simulink model "Simulation_invdyn"  (R2022b)
settings: Solver=ode1  StartTime=0.0  StopTime=Tf  FixedStep=t_step  RelTol=1e-3
undefined symbols (not defined in the file or in its folder): F, Im, Kd, Kp, kr, lx, ly, lz, mm, qt, rho, t_step
settings Model: Creator=vincenzo  LastModifiedBy=vincenzo

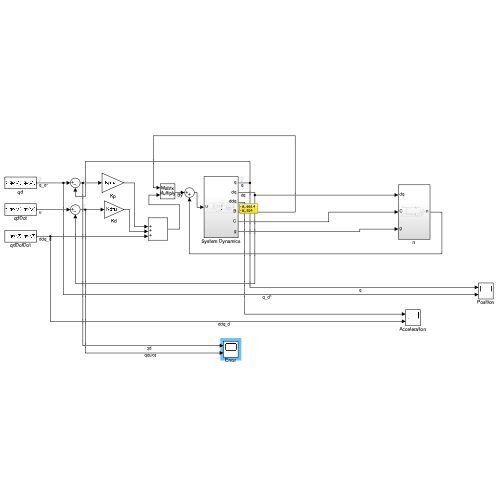
[thumbnail: Simulink's stored preview of the top-level diagram]
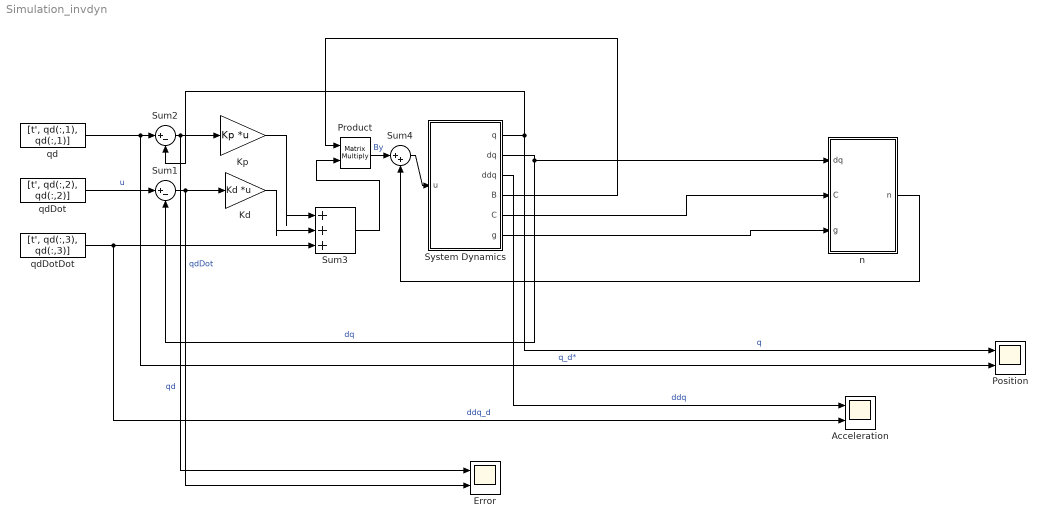
== system Simulation_invdyn ==
  Acceleration : Scope  NumInputPorts=2
  Error : Scope  NumInputPorts=2
  Kd : Gain  Gain=Kd  Multiplication=Matrix(K*u)
  Kp : Gain  Gain=Kp  Multiplication=Matrix(K*u)
  Position : Scope  NumInputPorts=2
  Product : Product  Multiplication=Matrix(*)
  Sum1 : Sum  Inputs=|+-
  Sum2 : Sum  Inputs=|+-
  Sum3 : Sum  Inputs=|+++
  Sum4 : Sum  Inputs=|++
  System Dynamics : Subsystem
  n : Subsystem
  qd : FromWorkspace  VariableName=[t', qd(:,1), qd(:,1)]  OutDataTypeStr=double  SampleTime=t_step
  qdDot : FromWorkspace  VariableName=[t', qd(:,2), qd(:,2)]  OutDataTypeStr=double  SampleTime=t_step
  qdDotDot : FromWorkspace  VariableName=[t', qd(:,3), qd(:,3)]  OutDataTypeStr=double  SampleTime=t_step
  wires:
  System Dynamics/2(dq) -> Sum1/2, n/1(dq)  "dq"
  System Dynamics/4(B) -> Product/1
  System Dynamics/5(C) -> n/2(C)
  System Dynamics/6(g) -> n/3(g)
  qd/1 -> Position/2, Sum2/1  "q_d*"
  Sum2/1 -> Error/1, Kp/1  "qd"
  qdDot/1 -> Sum1/1  "u"
  Sum1/1 -> Error/2, Kd/1  "qdDot"
  System Dynamics/1(q) -> Position/1, Sum2/2  "q"
  Kp/1 -> Sum3/1
  Kd/1 -> Sum3/2
  qdDotDot/1 -> Acceleration/2, Sum3/3  "ddq_d"
  Sum3/1 -> Product/2
  Product/1 -> Sum4/1  "By"
  Sum4/1 -> System Dynamics/1(u)
  n/1(n) -> Sum4/2
  System Dynamics/3(ddq) -> Acceleration/1  "ddq"

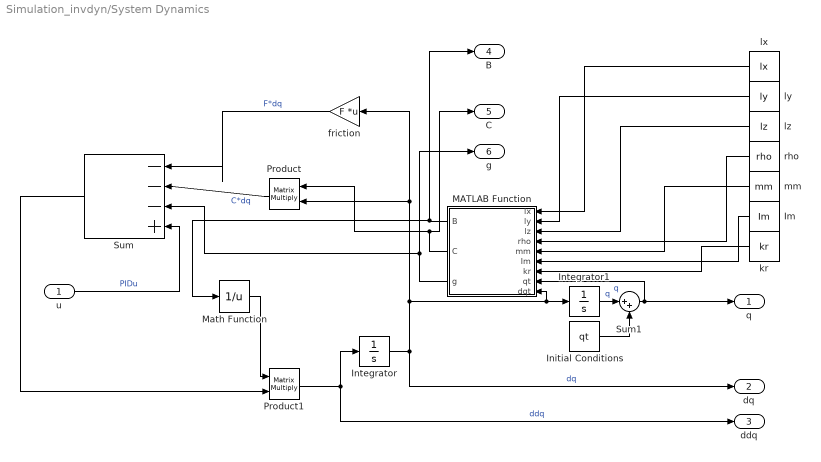
== system Simulation_invdyn/System Dynamics ==
  u : Inport
  Im : Constant  Value=Im
  Initial Conditions : Constant  Value=qt
  Integrator : Integrator  InitialCondition=[0; 0]
  Integrator1 : Integrator  InitialCondition=[0;0]
  MATLAB Function : MATLAB Function  TreatAsAtomicUnit=on
  Math Function : Math  Operator=reciprocal
  Product : Product  Multiplication=Matrix(*)
  Product1 : Product  Multiplication=Matrix(*)
  Sum : Sum  Inputs=|---+
  Sum1 : Sum  Inputs=|++
  friction : Gain  Gain=F  Multiplication=Matrix(K*u)
  kr : Constant  Value=kr
  lx : Constant  Value=lx
  ly : Constant  Value=ly
  lz : Constant  Value=lz
  mm : Constant  Value=mm
  rho : Constant  Value=rho
  q : Outport
  dq : Outport  Port=2
  ddq : Outport  Port=3
  B : Outport  Port=4
  C : Outport  Port=5
  g : Outport  Port=6
  wires:
  Sum/1 -> Product1/2
  friction/1 -> Sum/1  "F*dq"
  MATLAB Function/1(B) -> B/1, Math Function/1
  Sum1/1 -> MATLAB Function/8(qt), q/1  "q"
  lx/1 -> MATLAB Function/1(lx)
  MATLAB Function/2(C) -> C/1, Product/1
  Product/1 -> Sum/2  "C*dq"
  Math Function/1 -> Product1/1
  ly/1 -> MATLAB Function/2(ly)
  Integrator/1 -> Integrator1/1, MATLAB Function/9(dqt), Product/2, friction/1, dq/1  "dq"
  Product1/1 -> Integrator/1, ddq/1  "ddq"
  MATLAB Function/3(g) -> g/1, Sum/3
  lz/1 -> MATLAB Function/3(lz)
  mm/1 -> MATLAB Function/5(mm)
  kr/1 -> MATLAB Function/7(kr)
  rho/1 -> MATLAB Function/4(rho)
  Im/1 -> MATLAB Function/6(Im)
  u/1 -> Sum/4  "PIDu"
  Integrator1/1 -> Sum1/1  "q"
  Initial Conditions/1 -> Sum1/2

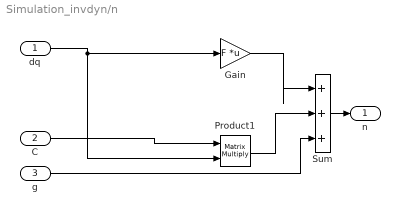
== system Simulation_invdyn/n ==
  dq : Inport
  C : Inport  Port=2
  g : Inport  Port=3
  Gain : Gain  Gain=F  Multiplication=Matrix(K*u)
  Product1 : Product  Multiplication=Matrix(*)
  Sum : Sum  Inputs=|+++
  n : Outport
  wires:
  g/1 -> Sum/3
  Sum/1 -> n/1
  Gain/1 -> Sum/1
  C/1 -> Product1/1
  dq/1 -> Product1/2, Gain/1
  Product1/1 -> Sum/2

== matlab function Simulation_invdyn/System Dynamics/MATLAB Function ==
  data: lx input; ly input; lz input; rho input; mm input; Im input; kr input; qt input; B output; dqt input; C output; g output
function [B, C, g] = fcn(lx, ly, lz, rho, mm, Im, kr, qt, dqt)
coder.extrinsic('generateBCg');
B = zeros(2);
C = zeros(2);
g = zeros(2,1);
[B, C, g] = generateBCg(lx, ly, lz, rho, mm, Im, kr, qt, dqt);
